simulink model "Robust_Adaptive_Control"  (R2015a)
settings: Solver=ode45  StartTime=0.0  StopTime=10  FixedStep=1e-3
libraries: aerolibutil x16, aerolibtransform2 x6, dspmtrx3 x6, simulink x1
(part 2 of 3)

== system Robust_Adaptive_Control/Slotine/u0-gen ==
  S : Inport
  sigma(t) : Inport  Port=2
  Divide : Product  Inputs=*/
  Dot Product : DotProduct  InputSameDT=on  OutDataTypeStr=Inherit: Inherit via internal rule
  Gain : Gain  Gain=-1
  Product : Product
  Product1 : Product
  Product2 : Product
  Sqrt : Sqrt  SaturateOnIntegerOverflow=on
  Sum : Sum  Inputs=|++
  gamma_hat : Integrator  InitialCondition=1
  u0 : Outport
  wires:
  gamma_hat/1 -> Product2/1, Product/2, Product/1
  Dot Product/1 -> Sqrt/1
  S/1 -> Product1/2, Dot Product/2, Dot Product/1
  Sqrt/1 -> Product2/2, gamma_hat/1
  Product/1 -> Product1/1
  Product1/1 -> Divide/1
  Product2/1 -> Sum/1
  Sum/1 -> Divide/2
  sigma(t)/1 -> Sum/2
  Divide/1 -> Gain/1
  Gain/1 -> u0/1

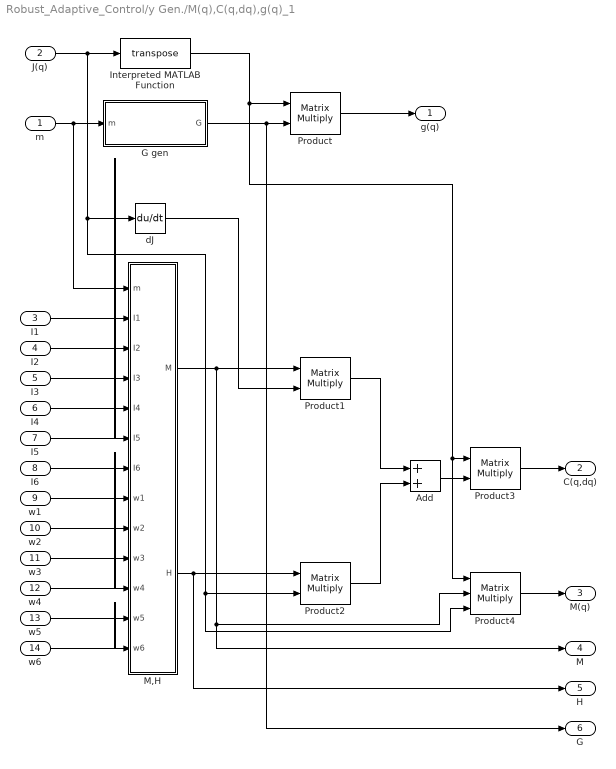
== system Robust_Adaptive_Control/y Gen./M(q),C(q,dq),g(q)_1 ==
  m : Inport
  J(q) : Inport  Port=2
  I1 : Inport  Port=3
  I2 : Inport  Port=4
  I3 : Inport  Port=5
  I4 : Inport  Port=6
  I5 : Inport  Port=7
  I6 : Inport  Port=8
  w1 : Inport  Port=9
  w2 : Inport  Port=10
  w3 : Inport  Port=11
  w4 : Inport  Port=12
  w5 : Inport  Port=13
  w6 : Inport  Port=14
  Add : Sum
  G gen : Subsystem
  Interpreted MATLAB Function : MATLABFcn  MATLABFcn=transpose  OutputSignalType=real  Output1D=off
  M,H : Subsystem
  Product{,1..3} (4 alike) : Product  Multiplication=Matrix(*)
  Product4 : Product  Inputs=3  Multiplication=Matrix(*)
  dJ : Derivative
  g(q) : Outport
  C(q,dq) : Outport  Port=2
  M(q) : Outport  Port=3
  M : Outport  Port=4
  H : Outport  Port=5
  G : Outport  Port=6
  wires:
  J(q)/1 -> Interpreted MATLAB Function/1, Product4/3, Product2/2, dJ/1
  Interpreted MATLAB Function/1 -> Product4/1, Product3/1, Product/1
  Product/1 -> g(q)/1
  m/1 -> M,H/1(m), G gen/1(m)
  I1/1 -> M,H/2(I1)
  I2/1 -> M,H/3(I2)
  I3/1 -> M,H/4(I3)
  I4/1 -> M,H/5(I4)
  I5/1 -> M,H/6(I5)
  I6/1 -> M,H/7(I6)
  w1/1 -> M,H/8(w1)
  w2/1 -> M,H/9(w2)
  w3/1 -> M,H/10(w3)
  w4/1 -> M,H/11(w4)
  w5/1 -> M,H/12(w5)
  w6/1 -> M,H/13(w6)
  M,H/1(M) -> Product1/1, M/1, Product4/2
  dJ/1 -> Product1/2
  M,H/2(H) -> H/1, Product2/1
  Product1/1 -> Add/1
  Product2/1 -> Add/2
  Add/1 -> Product3/2
  Product3/1 -> C(q,dq)/1
  Product4/1 -> M(q)/1
  G gen/1(G) -> G/1, Product/2

== system Robust_Adaptive_Control/y Gen./M(q),C(q,dq),g(q)_2 ==
  m : Inport
  J(q) : Inport  Port=2
  I1 : Inport  Port=3
  I2 : Inport  Port=4
  I3 : Inport  Port=5
  I4 : Inport  Port=6
  I5 : Inport  Port=7
  I6 : Inport  Port=8
  w1 : Inport  Port=9
  w2 : Inport  Port=10
  w3 : Inport  Port=11
  w4 : Inport  Port=12
  w5 : Inport  Port=13
  w6 : Inport  Port=14
  G gen : Subsystem
  Interpreted MATLAB Function : MATLABFcn  MATLABFcn=transpose  OutputSignalType=real  Output1D=off
  M,H : Subsystem
  Product : Product  Multiplication=Matrix(*)
  Product1 : Product  Multiplication=Matrix(*)
  Product3 : Product  Multiplication=Matrix(*)
  Product4 : Product  Inputs=3  Multiplication=Matrix(*)
  dJ : Derivative
  g(q) : Outport
  C(q,dq) : Outport  Port=2
  M(q) : Outport  Port=3
  M : Outport  Port=4
  H : Outport  Port=5
  G : Outport  Port=6
  wires:
  J(q)/1 -> Interpreted MATLAB Function/1, Product4/3, dJ/1
  Interpreted MATLAB Function/1 -> Product4/1, Product3/1, Product/1
  Product/1 -> g(q)/1
  m/1 -> G gen/1(m)
  I1/1 -> M,H/1(I1)
  I2/1 -> M,H/2(I2)
  I3/1 -> M,H/3(I3)
  I4/1 -> M,H/4(I4)
  I5/1 -> M,H/5(I5)
  I6/1 -> M,H/6(I6)
  w1/1 -> M,H/7(w1)
  w2/1 -> M,H/8(w2)
  w3/1 -> M,H/9(w3)
  w4/1 -> M,H/10(w4)
  w5/1 -> M,H/11(w5)
  w6/1 -> M,H/12(w6)
  M,H/1(M) -> Product1/1, M/1, Product4/2
  dJ/1 -> Product1/2
  M,H/2(H) -> H/1
  Product1/1 -> Product3/2
  Product3/1 -> C(q,dq)/1
  Product4/1 -> M(q)/1
  G gen/1(G) -> G/1, Product/2

== system Robust_Adaptive_Control/Jacobian/J(q) gen./J_v_1(q) ==
  Constant : Constant  Value=zeros(3,1)
  v2M_1 : MATLAB Function  TreatAsAtomicUnit=on
  v2M_2 : MATLAB Function  TreatAsAtomicUnit=on
  v2M_3 : MATLAB Function  TreatAsAtomicUnit=on
  v2M_4 : MATLAB Function  TreatAsAtomicUnit=on
  v2M_5 : MATLAB Function  TreatAsAtomicUnit=on
  J_v_1(q) : Outport
  wires:
  Constant/1 -> v2M_1/1(v1), v2M_5/2(v2), v2M_4/2(v2), v2M_3/2(v2), v2M_2/2(v2), v2M_1/2(v2)
  v2M_1/1(M) -> v2M_2/1(v1)
  v2M_2/1(M) -> v2M_3/1(v1)
  v2M_3/1(M) -> v2M_4/1(v1)
  v2M_4/1(M) -> v2M_5/1(v1)
  v2M_5/1(M) -> J_v_1(q)/1

== system Robust_Adaptive_Control/Jacobian/J(q) gen./J_v_2(q) ==
  R_1^0 : Inport
  p_1^0 : Inport  Port=2
  p_2^0 : Inport  Port=3
  type1 : Inport  Port=4
  Constant : Constant  Value=zeros(3,1)
  J_v_1 : Subsystem
  v2M_1 : MATLAB Function  TreatAsAtomicUnit=on
  v2M_2 : MATLAB Function  TreatAsAtomicUnit=on
  v2M_3 : MATLAB Function  TreatAsAtomicUnit=on
  v2M_4 : MATLAB Function  TreatAsAtomicUnit=on
  v2M_5 : MATLAB Function  TreatAsAtomicUnit=on
  J_v_2(q) : Outport
  wires:
  R_1^0/1 -> J_v_1/1(R)
  J_v_1/1(J_v) -> v2M_1/1(v1)
  v2M_1/1(M) -> v2M_2/1(v1)
  v2M_2/1(M) -> v2M_3/1(v1)
  v2M_3/1(M) -> v2M_4/1(v1)
  v2M_4/1(M) -> v2M_5/1(v1)
  v2M_5/1(M) -> J_v_2(q)/1
  Constant/1 -> v2M_3/2(v2), v2M_4/2(v2), v2M_5/2(v2), v2M_1/2(v2), v2M_2/2(v2)
  p_1^0/1 -> J_v_1/2(p)
  type1/1 -> J_v_1/4(type)
  p_2^0/1 -> J_v_1/3(pn)

== system Robust_Adaptive_Control/Jacobian/J(q) gen./J_v_3(q) ==
  R_1^0 : Inport
  R_2^0 : Inport  Port=2
  p_1^0 : Inport  Port=3
  p_2^0 : Inport  Port=4
  p_3^0 : Inport  Port=5
  type1 : Inport  Port=6
  type2 : Inport  Port=7
  Constant : Constant  Value=zeros(3,1)
  J_v_1 : Subsystem
  J_v_2 : Subsystem
  v2M_1 : MATLAB Function  TreatAsAtomicUnit=on
  v2M_2 : MATLAB Function  TreatAsAtomicUnit=on
  v2M_3 : MATLAB Function  TreatAsAtomicUnit=on
  v2M_4 : MATLAB Function  TreatAsAtomicUnit=on
  v2M_5 : MATLAB Function  TreatAsAtomicUnit=on
  J_v_3(q) : Outport
  wires:
  R_1^0/1 -> J_v_1/1(R)
  J_v_1/1(J_v) -> v2M_1/1(v1)
  v2M_1/1(M) -> v2M_2/1(v1)
  v2M_2/1(M) -> v2M_3/1(v1)
  v2M_3/1(M) -> v2M_4/1(v1)
  v2M_4/1(M) -> v2M_5/1(v1)
  v2M_5/1(M) -> J_v_3(q)/1
  J_v_2/1(J_v) -> v2M_1/2(v2)
  Constant/1 -> v2M_5/2(v2), v2M_4/2(v2), v2M_2/2(v2), v2M_3/2(v2)
  R_2^0/1 -> J_v_2/1(R)
  p_1^0/1 -> J_v_1/2(p)
  p_2^0/1 -> J_v_2/2(p)
  type2/1 -> J_v_2/4(type)
  type1/1 -> J_v_1/4(type)
  p_3^0/1 -> J_v_1/3(pn), J_v_2/3(pn)

== system Robust_Adaptive_Control/Jacobian/J(q) gen./J_v_4(q) ==
  R_1^0 : Inport
  R_2^0 : Inport  Port=2
  R_3^0 : Inport  Port=3
  p_1^0 : Inport  Port=4
  p_2^0 : Inport  Port=5
  p_3^0 : Inport  Port=6
  p_4^0 : Inport  Port=7
  type1 : Inport  Port=8
  type2 : Inport  Port=9
  type3 : Inport  Port=10
  Constant : Constant  Value=zeros(3,1)
  J_v_1 : Subsystem
  J_v_2 : Subsystem
  J_v_3 : Subsystem
  v2M_1 : MATLAB Function  TreatAsAtomicUnit=on
  v2M_2 : MATLAB Function  TreatAsAtomicUnit=on
  v2M_3 : MATLAB Function  TreatAsAtomicUnit=on
  v2M_4 : MATLAB Function  TreatAsAtomicUnit=on
  v2M_5 : MATLAB Function  TreatAsAtomicUnit=on
  J_v_4(q) : Outport
  wires:
  R_1^0/1 -> J_v_1/1(R)
  J_v_1/1(J_v) -> v2M_1/1(v1)
  v2M_1/1(M) -> v2M_2/1(v1)
  v2M_2/1(M) -> v2M_3/1(v1)
  v2M_3/1(M) -> v2M_4/1(v1)
  v2M_4/1(M) -> v2M_5/1(v1)
  v2M_5/1(M) -> J_v_4(q)/1
  J_v_2/1(J_v) -> v2M_1/2(v2)
  J_v_3/1(J_v) -> v2M_2/2(v2)
  Constant/1 -> v2M_5/2(v2), v2M_3/2(v2), v2M_4/2(v2)
  R_2^0/1 -> J_v_2/1(R)
  R_3^0/1 -> J_v_3/1(R)
  p_1^0/1 -> J_v_1/2(p)
  p_2^0/1 -> J_v_2/2(p)
  p_3^0/1 -> J_v_3/2(p)
  type2/1 -> J_v_2/4(type)
  type1/1 -> J_v_1/4(type)
  type3/1 -> J_v_3/4(type)
  p_4^0/1 -> J_v_1/3(pn), J_v_2/3(pn), J_v_3/3(pn)

== system Robust_Adaptive_Control/Jacobian/J(q) gen./J_v_5(q) ==
  R_1^0 : Inport
  R_2^0 : Inport  Port=2
  R_3^0 : Inport  Port=3
  R_4^0 : Inport  Port=4
  p_1^0 : Inport  Port=5
  p_2^0 : Inport  Port=6
  p_3^0 : Inport  Port=7
  p_4^0 : Inport  Port=8
  p_5^0 : Inport  Port=9
  type1 : Inport  Port=10
  type2 : Inport  Port=11
  type3 : Inport  Port=12
  type4 : Inport  Port=13
  Constant : Constant  Value=zeros(3,1)
  J_v_1 : Subsystem
  J_v_2 : Subsystem
  J_v_3 : Subsystem
  J_v_4 : Subsystem
  v2M_1 : MATLAB Function  TreatAsAtomicUnit=on
  v2M_2 : MATLAB Function  TreatAsAtomicUnit=on
  v2M_3 : MATLAB Function  TreatAsAtomicUnit=on
  v2M_4 : MATLAB Function  TreatAsAtomicUnit=on
  v2M_5 : MATLAB Function  TreatAsAtomicUnit=on
  J_v_5(q) : Outport
  wires:
  R_1^0/1 -> J_v_1/1(R)
  J_v_1/1(J_v) -> v2M_1/1(v1)
  v2M_1/1(M) -> v2M_2/1(v1)
  v2M_2/1(M) -> v2M_3/1(v1)
  v2M_3/1(M) -> v2M_4/1(v1)
  v2M_4/1(M) -> v2M_5/1(v1)
  v2M_5/1(M) -> J_v_5(q)/1
  J_v_2/1(J_v) -> v2M_1/2(v2)
  J_v_3/1(J_v) -> v2M_2/2(v2)
  J_v_4/1(J_v) -> v2M_3/2(v2)
  Constant/1 -> v2M_4/2(v2), v2M_5/2(v2)
  R_2^0/1 -> J_v_2/1(R)
  R_3^0/1 -> J_v_3/1(R)
  R_4^0/1 -> J_v_4/1(R)
  p_1^0/1 -> J_v_1/2(p)
  p_2^0/1 -> J_v_2/2(p)
  p_3^0/1 -> J_v_3/2(p)
  p_4^0/1 -> J_v_4/2(p)
  type2/1 -> J_v_2/4(type)
  type1/1 -> J_v_1/4(type)
  type3/1 -> J_v_3/4(type)
  type4/1 -> J_v_4/4(type)
  p_5^0/1 -> J_v_1/3(pn), J_v_2/3(pn), J_v_3/3(pn), J_v_4/3(pn)

== system Robust_Adaptive_Control/Jacobian/J_v/J_v_1 ==
  R : Inport
  p : Inport  Port=2
  pn : Inport  Port=3
  type : Inport  Port=4
  Add : Sum
  If : If  IfExpression=u1 == 1
  Prismatic Action : Subsystem  TreatAsAtomicUnit=on
  Revolute Action : Subsystem  TreatAsAtomicUnit=on
  J_v : Outport
  wires:
  type/1 -> If/1
  If/1 -> Revolute Action/Action
  If/2 -> Prismatic Action/Action
  Revolute Action/1(J_v) -> Add/1
  Prismatic Action/1(J_v) -> Add/2
  Add/1 -> J_v/1
  R/1 -> Prismatic Action/1(R), Revolute Action/1(R)
  p/1 -> Revolute Action/2(p)
  pn/1 -> Revolute Action/3(pn)

== system Robust_Adaptive_Control/Jacobian/J_v/J_v_2 ==
  R : Inport
  p : Inport  Port=2
  pn : Inport  Port=3
  type : Inport  Port=4
  Add : Sum
  If : If  IfExpression=u1 == 1
  Prismatic Action : Subsystem  TreatAsAtomicUnit=on
  Revolute Action : Subsystem  TreatAsAtomicUnit=on
  J_v : Outport
  wires:
  type/1 -> If/1
  If/1 -> Revolute Action/Action
  If/2 -> Prismatic Action/Action
  Revolute Action/1(J_v) -> Add/1
  Prismatic Action/1(J_v) -> Add/2
  Add/1 -> J_v/1
  R/1 -> Prismatic Action/1(R), Revolute Action/1(R)
  p/1 -> Revolute Action/2(p)
  pn/1 -> Revolute Action/3(pn)

== system Robust_Adaptive_Control/Jacobian/J_v/J_v_3 ==
  R : Inport
  p : Inport  Port=2
  pn : Inport  Port=3
  type : Inport  Port=4
  Add : Sum
  If : If  IfExpression=u1 == 1
  Prismatic Action : Subsystem  TreatAsAtomicUnit=on
  Revolute Action : Subsystem  TreatAsAtomicUnit=on
  J_v : Outport
  wires:
  type/1 -> If/1
  If/1 -> Revolute Action/Action
  If/2 -> Prismatic Action/Action
  Revolute Action/1(J_v) -> Add/1
  Prismatic Action/1(J_v) -> Add/2
  Add/1 -> J_v/1
  R/1 -> Prismatic Action/1(R), Revolute Action/1(R)
  p/1 -> Revolute Action/2(p)
  pn/1 -> Revolute Action/3(pn)

== system Robust_Adaptive_Control/Jacobian/J_v/J_v_4 ==
  R : Inport
  p : Inport  Port=2
  pn : Inport  Port=3
  type : Inport  Port=4
  Add : Sum
  If : If  IfExpression=u1 == 1
  Prismatic Action : Subsystem  TreatAsAtomicUnit=on
  Revolute Action : Subsystem  TreatAsAtomicUnit=on
  J_v : Outport
  wires:
  type/1 -> If/1
  If/1 -> Revolute Action/Action
  If/2 -> Prismatic Action/Action
  Revolute Action/1(J_v) -> Add/1
  Prismatic Action/1(J_v) -> Add/2
  Add/1 -> J_v/1
  R/1 -> Prismatic Action/1(R), Revolute Action/1(R)
  p/1 -> Revolute Action/2(p)
  pn/1 -> Revolute Action/3(pn)

== system Robust_Adaptive_Control/Jacobian/J_v/J_v_5 ==
  R : Inport
  p : Inport  Port=2
  pn : Inport  Port=3
  type : Inport  Port=4
  Add : Sum
  If : If  IfExpression=u1 == 1
  Prismatic Action : Subsystem  TreatAsAtomicUnit=on
  Revolute Action : Subsystem  TreatAsAtomicUnit=on
  J_v : Outport
  wires:
  type/1 -> If/1
  If/1 -> Revolute Action/Action
  If/2 -> Prismatic Action/Action
  Revolute Action/1(J_v) -> Add/1
  Prismatic Action/1(J_v) -> Add/2
  Add/1 -> J_v/1
  R/1 -> Prismatic Action/1(R), Revolute Action/1(R)
  p/1 -> Revolute Action/2(p)
  pn/1 -> Revolute Action/3(pn)

== system Robust_Adaptive_Control/Jacobian/J_v/J_v_6 ==
  R : Inport
  p : Inport  Port=2
  pn : Inport  Port=3
  type : Inport  Port=4
  Add : Sum
  If : If  IfExpression=u1 == 1
  Prismatic Action : Subsystem  TreatAsAtomicUnit=on
  Revolute Action : Subsystem  TreatAsAtomicUnit=on
  J_v : Outport
  wires:
  type/1 -> If/1
  If/1 -> Revolute Action/Action
  If/2 -> Prismatic Action/Action
  Revolute Action/1(J_v) -> Add/1
  Prismatic Action/1(J_v) -> Add/2
  Add/1 -> J_v/1
  R/1 -> Prismatic Action/1(R), Revolute Action/1(R)
  p/1 -> Revolute Action/2(p)
  pn/1 -> Revolute Action/3(pn)

== system Robust_Adaptive_Control/y Gen./M(q),C(q,dq),g(q)_1/G gen ==
  m : Inport
  Demux : Demux  Outputs=6
  Mux : Mux  Inputs=7
  Product{,1..5} (6 alike) : Product
  g : Constant  Value=[0;0;9.81]
  g1 : Constant  Value=zeros(18,1)
  G : Outport
  wires:
  m/1 -> Demux/1
  Demux/1 -> Product/1
  Demux/2 -> Product1/1
  Demux/3 -> Product2/1
  g/1 -> Product5/2, Product4/2, Product3/2, Product2/2, Product1/2, Product/2
  Demux/4 -> Product3/1
  Demux/5 -> Product4/1
  Demux/6 -> Product5/1
  Product1/1 -> Mux/2
  Product/1 -> Mux/1
  Product2/1 -> Mux/3
  Product4/1 -> Mux/5
  Product5/1 -> Mux/6
  Product3/1 -> Mux/4
  g1/1 -> Mux/7
  Mux/1 -> G/1

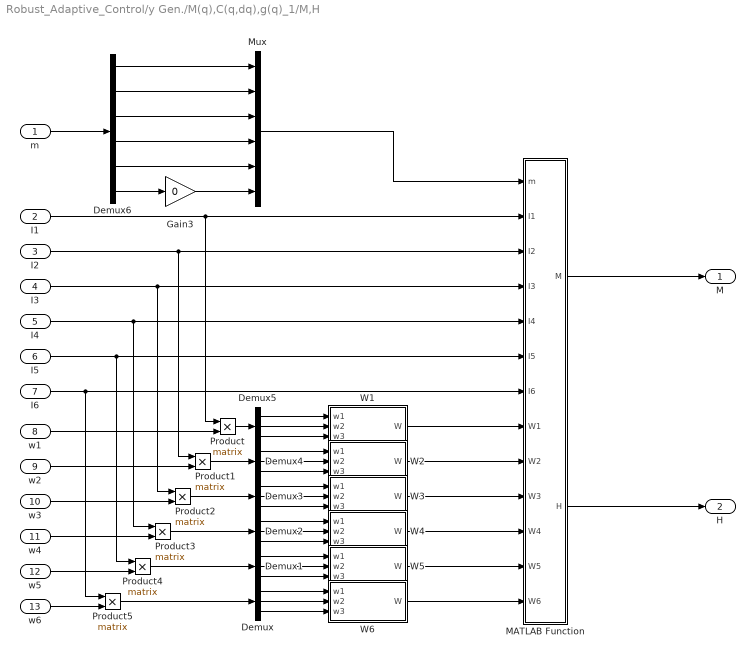
== system Robust_Adaptive_Control/y Gen./M(q),C(q,dq),g(q)_1/M,H ==
  m : Inport
  I1 : Inport  Port=2
  I2 : Inport  Port=3
  I3 : Inport  Port=4
  I4 : Inport  Port=5
  I5 : Inport  Port=6
  I6 : Inport  Port=7
  w1 : Inport  Port=8
  w2 : Inport  Port=9
  w3 : Inport  Port=10
  w4 : Inport  Port=11
  w5 : Inport  Port=12
  w6 : Inport  Port=13
  Demux{,1..5} (6 alike) : Demux  Outputs=3
  Demux6 : Demux  Outputs=6
  Gain3 : Gain  Gain=0
  MATLAB Function : MATLAB Function  TreatAsAtomicUnit=on
  Mux : Mux  Inputs=6
  Product{,1..5} (6 alike) : Product  Multiplication=Matrix(*)
  W1 : MATLAB Function  TreatAsAtomicUnit=on
  W2 : MATLAB Function  TreatAsAtomicUnit=on
  W3 : MATLAB Function  TreatAsAtomicUnit=on
  W4 : MATLAB Function  TreatAsAtomicUnit=on
  W5 : MATLAB Function  TreatAsAtomicUnit=on
  W6 : MATLAB Function  TreatAsAtomicUnit=on
  M : Outport
  H : Outport  Port=2
  wires:
  I1/1 -> Product/1, MATLAB Function/2(I1)
  I2/1 -> Product1/1, MATLAB Function/3(I2)
  I3/1 -> Product2/1, MATLAB Function/4(I3)
  I4/1 -> Product3/1, MATLAB Function/5(I4)
  I5/1 -> Product4/1, MATLAB Function/6(I5)
  I6/1 -> Product5/1, MATLAB Function/7(I6)
  MATLAB Function/1(M) -> M/1
  MATLAB Function/2(H) -> H/1
  W1/1(W) -> MATLAB Function/8(W1)
  W2/1(W) -> MATLAB Function/9(W2)
  W3/1(W) -> MATLAB Function/10(W3)
  W4/1(W) -> MATLAB Function/11(W4)
  W5/1(W) -> MATLAB Function/12(W5)
  W6/1(W) -> MATLAB Function/13(W6)
  w6/1 -> Product5/2
  Demux/3 -> W6/3(w3)
  Demux/2 -> W6/2(w2)
  Demux/1 -> W6/1(w1)
  w5/1 -> Product4/2
  Demux1/3 -> W5/3(w3)
  Demux1/2 -> W5/2(w2)
  Demux1/1 -> W5/1(w1)
  w4/1 -> Product3/2
  Demux2/3 -> W4/3(w3)
  Demux2/2 -> W4/2(w2)
  Demux2/1 -> W4/1(w1)
  w3/1 -> Product2/2
  Demux3/3 -> W3/3(w3)
  Demux3/2 -> W3/2(w2)
  Demux3/1 -> W3/1(w1)
  w2/1 -> Product1/2
  Demux4/3 -> W2/3(w3)
  Demux4/2 -> W2/2(w2)
  Demux4/1 -> W2/1(w1)
  w1/1 -> Product/2
  Demux5/3 -> W1/3(w3)
  Demux5/2 -> W1/2(w2)
  Demux5/1 -> W1/1(w1)
  Product/1 -> Demux5/1
  Product1/1 -> Demux4/1
  Product2/1 -> Demux3/1
  Product3/1 -> Demux2/1
  Product4/1 -> Demux1/1
  Product5/1 -> Demux/1
  m/1 -> Demux6/1
  Mux/1 -> MATLAB Function/1(m)
  Demux6/2 -> Mux/2
  Demux6/3 -> Mux/3
  Demux6/4 -> Mux/4
  Demux6/5 -> Mux/5
  Demux6/1 -> Mux/1
  Demux6/6 -> Gain3/1
  Gain3/1 -> Mux/6

== system Robust_Adaptive_Control/y Gen./M(q),C(q,dq),g(q)_2/G gen ==
  m : Inport
  Demux : Demux  Outputs=6
  Mux : Mux  Inputs=7
  Product{,1..5} (6 alike) : Product
  g : Constant  Value=[0;0;9.81]
  g1 : Constant  Value=zeros(18,1)
  G : Outport
  wires:
  m/1 -> Demux/1
  Demux/1 -> Product/1
  Demux/2 -> Product1/1
  Demux/3 -> Product2/1
  g/1 -> Product5/2, Product4/2, Product3/2, Product2/2, Product1/2, Product/2
  Demux/4 -> Product3/1
  Demux/5 -> Product4/1
  Demux/6 -> Product5/1
  Product1/1 -> Mux/2
  Product/1 -> Mux/1
  Product2/1 -> Mux/3
  Product4/1 -> Mux/5
  Product5/1 -> Mux/6
  Product3/1 -> Mux/4
  g1/1 -> Mux/7
  Mux/1 -> G/1

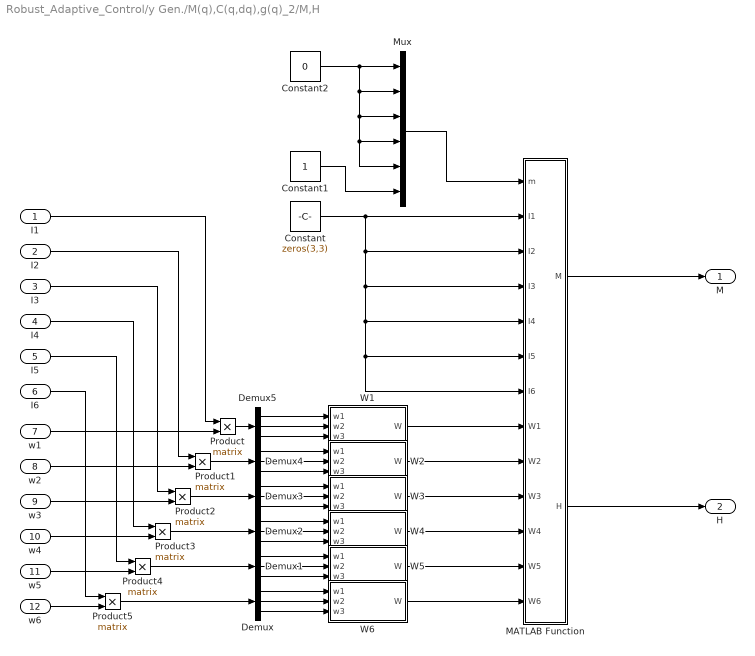
== system Robust_Adaptive_Control/y Gen./M(q),C(q,dq),g(q)_2/M,H ==
  I1 : Inport
  I2 : Inport  Port=2
  I3 : Inport  Port=3
  I4 : Inport  Port=4
  I5 : Inport  Port=5
  I6 : Inport  Port=6
  w1 : Inport  Port=7
  w2 : Inport  Port=8
  w3 : Inport  Port=9
  w4 : Inport  Port=10
  w5 : Inport  Port=11
  w6 : Inport  Port=12
  Constant : Constant  Value=zeros(3,3)
  Constant1 : Constant
  Constant2 : Constant  Value=0
  Demux{,1..5} (6 alike) : Demux  Outputs=3
  MATLAB Function : MATLAB Function  TreatAsAtomicUnit=on
  Mux : Mux  Inputs=6
  Product{,1..5} (6 alike) : Product  Multiplication=Matrix(*)
  W1 : MATLAB Function  TreatAsAtomicUnit=on
  W2 : MATLAB Function  TreatAsAtomicUnit=on
  W3 : MATLAB Function  TreatAsAtomicUnit=on
  W4 : MATLAB Function  TreatAsAtomicUnit=on
  W5 : MATLAB Function  TreatAsAtomicUnit=on
  W6 : MATLAB Function  TreatAsAtomicUnit=on
  M : Outport
  H : Outport  Port=2
  wires:
  I1/1 -> Product/1
  I2/1 -> Product1/1
  I3/1 -> Product2/1
  I4/1 -> Product3/1
  I5/1 -> Product4/1
  I6/1 -> Product5/1
  MATLAB Function/1(M) -> M/1
  MATLAB Function/2(H) -> H/1
  W1/1(W) -> MATLAB Function/8(W1)
  W2/1(W) -> MATLAB Function/9(W2)
  W3/1(W) -> MATLAB Function/10(W3)
  W4/1(W) -> MATLAB Function/11(W4)
  W5/1(W) -> MATLAB Function/12(W5)
  W6/1(W) -> MATLAB Function/13(W6)
  w6/1 -> Product5/2
  Demux/3 -> W6/3(w3)
  Demux/2 -> W6/2(w2)
  Demux/1 -> W6/1(w1)
  w5/1 -> Product4/2
  Demux1/3 -> W5/3(w3)
  Demux1/2 -> W5/2(w2)
  Demux1/1 -> W5/1(w1)
  w4/1 -> Product3/2
  Demux2/3 -> W4/3(w3)
  Demux2/2 -> W4/2(w2)
  Demux2/1 -> W4/1(w1)
  w3/1 -> Product2/2
  Demux3/3 -> W3/3(w3)
  Demux3/2 -> W3/2(w2)
  Demux3/1 -> W3/1(w1)
  w2/1 -> Product1/2
  Demux4/3 -> W2/3(w3)
  Demux4/2 -> W2/2(w2)
  Demux4/1 -> W2/1(w1)
  w1/1 -> Product/2
  Demux5/3 -> W1/3(w3)
  Demux5/2 -> W1/2(w2)
  Demux5/1 -> W1/1(w1)
  Product/1 -> Demux5/1
  Product1/1 -> Demux4/1
  Product2/1 -> Demux3/1
  Product3/1 -> Demux2/1
  Product4/1 -> Demux1/1
  Product5/1 -> Demux/1
  Mux/1 -> MATLAB Function/1(m)
  Constant/1 -> MATLAB Function/7(I6), MATLAB Function/6(I5), MATLAB Function/5(I4), MATLAB Function/4(I3), MATLAB Function/3(I2), MATLAB Function/2(I1)
  Constant1/1 -> Mux/6
  Constant2/1 -> Mux/3, Mux/5, Mux/4, Mux/2, Mux/1

== system Robust_Adaptive_Control/Jacobian/J(q) gen./J_v_2(q)/J_v_1 ==
  R : Inport
  p : Inport  Port=2
  pn : Inport  Port=3
  type : Inport  Port=4
  Add : Sum
  If : If  IfExpression=u1 == 1
  Prismatic Action : Subsystem  TreatAsAtomicUnit=on
  Revolute Action : Subsystem  TreatAsAtomicUnit=on
  J_v : Outport
  wires:
  type/1 -> If/1
  If/1 -> Revolute Action/Action
  If/2 -> Prismatic Action/Action
  Revolute Action/1(J_v) -> Add/1
  Prismatic Action/1(J_v) -> Add/2
  Add/1 -> J_v/1
  R/1 -> Prismatic Action/1(R), Revolute Action/1(R)
  p/1 -> Revolute Action/2(p)
  pn/1 -> Revolute Action/3(pn)

== system Robust_Adaptive_Control/Jacobian/J(q) gen./J_v_3(q)/J_v_1 ==
  R : Inport
  p : Inport  Port=2
  pn : Inport  Port=3
  type : Inport  Port=4
  Add : Sum
  If : If  IfExpression=u1 == 1
  Prismatic Action : Subsystem  TreatAsAtomicUnit=on
  Revolute Action : Subsystem  TreatAsAtomicUnit=on
  J_v : Outport
  wires:
  type/1 -> If/1
  If/1 -> Revolute Action/Action
  If/2 -> Prismatic Action/Action
  Revolute Action/1(J_v) -> Add/1
  Prismatic Action/1(J_v) -> Add/2
  Add/1 -> J_v/1
  R/1 -> Prismatic Action/1(R), Revolute Action/1(R)
  p/1 -> Revolute Action/2(p)
  pn/1 -> Revolute Action/3(pn)

== system Robust_Adaptive_Control/Jacobian/J(q) gen./J_v_3(q)/J_v_2 ==
  R : Inport
  p : Inport  Port=2
  pn : Inport  Port=3
  type : Inport  Port=4
  Add : Sum
  If : If  IfExpression=u1 == 1
  Prismatic Action : Subsystem  TreatAsAtomicUnit=on
  Revolute Action : Subsystem  TreatAsAtomicUnit=on
  J_v : Outport
  wires:
  type/1 -> If/1
  If/1 -> Revolute Action/Action
  If/2 -> Prismatic Action/Action
  Revolute Action/1(J_v) -> Add/1
  Prismatic Action/1(J_v) -> Add/2
  Add/1 -> J_v/1
  R/1 -> Prismatic Action/1(R), Revolute Action/1(R)
  p/1 -> Revolute Action/2(p)
  pn/1 -> Revolute Action/3(pn)

== system Robust_Adaptive_Control/Jacobian/J(q) gen./J_v_4(q)/J_v_1 ==
  R : Inport
  p : Inport  Port=2
  pn : Inport  Port=3
  type : Inport  Port=4
  Add : Sum
  If : If  IfExpression=u1 == 1
  Prismatic Action : Subsystem  TreatAsAtomicUnit=on
  Revolute Action : Subsystem  TreatAsAtomicUnit=on
  J_v : Outport
  wires:
  type/1 -> If/1
  If/1 -> Revolute Action/Action
  If/2 -> Prismatic Action/Action
  Revolute Action/1(J_v) -> Add/1
  Prismatic Action/1(J_v) -> Add/2
  Add/1 -> J_v/1
  R/1 -> Prismatic Action/1(R), Revolute Action/1(R)
  p/1 -> Revolute Action/2(p)
  pn/1 -> Revolute Action/3(pn)

== system Robust_Adaptive_Control/Jacobian/J(q) gen./J_v_4(q)/J_v_2 ==
  R : Inport
  p : Inport  Port=2
  pn : Inport  Port=3
  type : Inport  Port=4
  Add : Sum
  If : If  IfExpression=u1 == 1
  Prismatic Action : Subsystem  TreatAsAtomicUnit=on
  Revolute Action : Subsystem  TreatAsAtomicUnit=on
  J_v : Outport
  wires:
  type/1 -> If/1
  If/1 -> Revolute Action/Action
  If/2 -> Prismatic Action/Action
  Revolute Action/1(J_v) -> Add/1
  Prismatic Action/1(J_v) -> Add/2
  Add/1 -> J_v/1
  R/1 -> Prismatic Action/1(R), Revolute Action/1(R)
  p/1 -> Revolute Action/2(p)
  pn/1 -> Revolute Action/3(pn)

== system Robust_Adaptive_Control/Jacobian/J(q) gen./J_v_4(q)/J_v_3 ==
  R : Inport
  p : Inport  Port=2
  pn : Inport  Port=3
  type : Inport  Port=4
  Add : Sum
  If : If  IfExpression=u1 == 1
  Prismatic Action : Subsystem  TreatAsAtomicUnit=on
  Revolute Action : Subsystem  TreatAsAtomicUnit=on
  J_v : Outport
  wires:
  type/1 -> If/1
  If/1 -> Revolute Action/Action
  If/2 -> Prismatic Action/Action
  Revolute Action/1(J_v) -> Add/1
  Prismatic Action/1(J_v) -> Add/2
  Add/1 -> J_v/1
  R/1 -> Prismatic Action/1(R), Revolute Action/1(R)
  p/1 -> Revolute Action/2(p)
  pn/1 -> Revolute Action/3(pn)

== system Robust_Adaptive_Control/Jacobian/J(q) gen./J_v_5(q)/J_v_1 ==
  R : Inport
  p : Inport  Port=2
  pn : Inport  Port=3
  type : Inport  Port=4
  Add : Sum
  If : If  IfExpression=u1 == 1
  Prismatic Action : Subsystem  TreatAsAtomicUnit=on
  Revolute Action : Subsystem  TreatAsAtomicUnit=on
  J_v : Outport
  wires:
  type/1 -> If/1
  If/1 -> Revolute Action/Action
  If/2 -> Prismatic Action/Action
  Revolute Action/1(J_v) -> Add/1
  Prismatic Action/1(J_v) -> Add/2
  Add/1 -> J_v/1
  R/1 -> Prismatic Action/1(R), Revolute Action/1(R)
  p/1 -> Revolute Action/2(p)
  pn/1 -> Revolute Action/3(pn)

== system Robust_Adaptive_Control/Jacobian/J(q) gen./J_v_5(q)/J_v_2 ==
  R : Inport
  p : Inport  Port=2
  pn : Inport  Port=3
  type : Inport  Port=4
  Add : Sum
  If : If  IfExpression=u1 == 1
  Prismatic Action : Subsystem  TreatAsAtomicUnit=on
  Revolute Action : Subsystem  TreatAsAtomicUnit=on
  J_v : Outport
  wires:
  type/1 -> If/1
  If/1 -> Revolute Action/Action
  If/2 -> Prismatic Action/Action
  Revolute Action/1(J_v) -> Add/1
  Prismatic Action/1(J_v) -> Add/2
  Add/1 -> J_v/1
  R/1 -> Prismatic Action/1(R), Revolute Action/1(R)
  p/1 -> Revolute Action/2(p)
  pn/1 -> Revolute Action/3(pn)

== system Robust_Adaptive_Control/Jacobian/J(q) gen./J_v_5(q)/J_v_3 ==
  R : Inport
  p : Inport  Port=2
  pn : Inport  Port=3
  type : Inport  Port=4
  Add : Sum
  If : If  IfExpression=u1 == 1
  Prismatic Action : Subsystem  TreatAsAtomicUnit=on
  Revolute Action : Subsystem  TreatAsAtomicUnit=on
  J_v : Outport
  wires:
  type/1 -> If/1
  If/1 -> Revolute Action/Action
  If/2 -> Prismatic Action/Action
  Revolute Action/1(J_v) -> Add/1
  Prismatic Action/1(J_v) -> Add/2
  Add/1 -> J_v/1
  R/1 -> Prismatic Action/1(R), Revolute Action/1(R)
  p/1 -> Revolute Action/2(p)
  pn/1 -> Revolute Action/3(pn)

== system Robust_Adaptive_Control/Jacobian/J(q) gen./J_v_5(q)/J_v_4 ==
  R : Inport
  p : Inport  Port=2
  pn : Inport  Port=3
  type : Inport  Port=4
  Add : Sum
  If : If  IfExpression=u1 == 1
  Prismatic Action : Subsystem  TreatAsAtomicUnit=on
  Revolute Action : Subsystem  TreatAsAtomicUnit=on
  J_v : Outport
  wires:
  type/1 -> If/1
  If/1 -> Revolute Action/Action
  If/2 -> Prismatic Action/Action
  Revolute Action/1(J_v) -> Add/1
  Prismatic Action/1(J_v) -> Add/2
  Add/1 -> J_v/1
  R/1 -> Prismatic Action/1(R), Revolute Action/1(R)
  p/1 -> Revolute Action/2(p)
  pn/1 -> Revolute Action/3(pn)

== system Robust_Adaptive_Control/Jacobian/J_v/J_v_1/Prismatic Action ==
  R : Inport
  Action Port : ActionPort  ActionType=else
  Constant : Constant  Value=[0;0;1]
  Product : Product  Multiplication=Matrix(*)
  J_v : Outport
  wires:
  Product/1 -> J_v/1
  R/1 -> Product/1
  Constant/1 -> Product/2

== system Robust_Adaptive_Control/Jacobian/J_v/J_v_1/Revolute Action ==
  R : Inport
  p : Inport  Port=2
  pn : Inport  Port=3
  Action Port : ActionPort  ActionType=then
  3x3 Cross Product : aerolibutil/3x3 Cross Product
  Add : Sum  Inputs=-+
  Constant : Constant  Value=[0;0;1]
  Product : Product  Multiplication=Matrix(*)
  J_v : Outport
  wires:
  3x3 Cross Product/1 -> J_v/1
  p/1 -> Add/1
  pn/1 -> Add/2
  Add/1 -> 3x3 Cross Product/2
  R/1 -> Product/1
  Constant/1 -> Product/2
  Product/1 -> 3x3 Cross Product/1

== system Robust_Adaptive_Control/Jacobian/J_v/J_v_2/Prismatic Action ==
  R : Inport
  Action Port : ActionPort  ActionType=else
  Constant : Constant  Value=[0;0;1]
  Product : Product  Multiplication=Matrix(*)
  J_v : Outport
  wires:
  Product/1 -> J_v/1
  R/1 -> Product/1
  Constant/1 -> Product/2

== system Robust_Adaptive_Control/Jacobian/J_v/J_v_2/Revolute Action ==
  R : Inport
  p : Inport  Port=2
  pn : Inport  Port=3
  Action Port : ActionPort  ActionType=then
  3x3 Cross Product : aerolibutil/3x3 Cross Product
  Add : Sum  Inputs=-+
  Constant : Constant  Value=[0;0;1]
  Product : Product  Multiplication=Matrix(*)
  J_v : Outport
  wires:
  3x3 Cross Product/1 -> J_v/1
  p/1 -> Add/1
  pn/1 -> Add/2
  Add/1 -> 3x3 Cross Product/2
  R/1 -> Product/1
  Constant/1 -> Product/2
  Product/1 -> 3x3 Cross Product/1

== system Robust_Adaptive_Control/Jacobian/J_v/J_v_3/Prismatic Action ==
  R : Inport
  Action Port : ActionPort  ActionType=else
  Constant : Constant  Value=[0;0;1]
  Product : Product  Multiplication=Matrix(*)
  J_v : Outport
  wires:
  Product/1 -> J_v/1
  R/1 -> Product/1
  Constant/1 -> Product/2

== system Robust_Adaptive_Control/Jacobian/J_v/J_v_3/Revolute Action ==
  R : Inport
  p : Inport  Port=2
  pn : Inport  Port=3
  Action Port : ActionPort  ActionType=then
  3x3 Cross Product : aerolibutil/3x3 Cross Product
  Add : Sum  Inputs=-+
  Constant : Constant  Value=[0;0;1]
  Product : Product  Multiplication=Matrix(*)
  J_v : Outport
  wires:
  3x3 Cross Product/1 -> J_v/1
  p/1 -> Add/1
  pn/1 -> Add/2
  Add/1 -> 3x3 Cross Product/2
  R/1 -> Product/1
  Constant/1 -> Product/2
  Product/1 -> 3x3 Cross Product/1

== system Robust_Adaptive_Control/Jacobian/J_v/J_v_4/Prismatic Action ==
  R : Inport
  Action Port : ActionPort  ActionType=else
  Constant : Constant  Value=[0;0;1]
  Product : Product  Multiplication=Matrix(*)
  J_v : Outport
  wires:
  Product/1 -> J_v/1
  R/1 -> Product/1
  Constant/1 -> Product/2

== system Robust_Adaptive_Control/Jacobian/J_v/J_v_4/Revolute Action ==
  R : Inport
  p : Inport  Port=2
  pn : Inport  Port=3
  Action Port : ActionPort  ActionType=then
  3x3 Cross Product : aerolibutil/3x3 Cross Product
  Add : Sum  Inputs=-+
  Constant : Constant  Value=[0;0;1]
  Product : Product  Multiplication=Matrix(*)
  J_v : Outport
  wires:
  3x3 Cross Product/1 -> J_v/1
  p/1 -> Add/1
  pn/1 -> Add/2
  Add/1 -> 3x3 Cross Product/2
  R/1 -> Product/1
  Constant/1 -> Product/2
  Product/1 -> 3x3 Cross Product/1

== system Robust_Adaptive_Control/Jacobian/J_v/J_v_5/Prismatic Action ==
  R : Inport
  Action Port : ActionPort  ActionType=else
  Constant : Constant  Value=[0;0;1]
  Product : Product  Multiplication=Matrix(*)
  J_v : Outport
  wires:
  Product/1 -> J_v/1
  R/1 -> Product/1
  Constant/1 -> Product/2

== system Robust_Adaptive_Control/Jacobian/J_v/J_v_5/Revolute Action ==
  R : Inport
  p : Inport  Port=2
  pn : Inport  Port=3
  Action Port : ActionPort  ActionType=then
  3x3 Cross Product : aerolibutil/3x3 Cross Product
  Add : Sum  Inputs=-+
  Constant : Constant  Value=[0;0;1]
  Product : Product  Multiplication=Matrix(*)
  J_v : Outport
  wires:
  3x3 Cross Product/1 -> J_v/1
  p/1 -> Add/1
  pn/1 -> Add/2
  Add/1 -> 3x3 Cross Product/2
  R/1 -> Product/1
  Constant/1 -> Product/2
  Product/1 -> 3x3 Cross Product/1

== system Robust_Adaptive_Control/Jacobian/J_v/J_v_6/Prismatic Action ==
  R : Inport
  Action Port : ActionPort  ActionType=else
  Constant : Constant  Value=[0;0;1]
  Product : Product  Multiplication=Matrix(*)
  J_v : Outport
  wires:
  Product/1 -> J_v/1
  R/1 -> Product/1
  Constant/1 -> Product/2

== system Robust_Adaptive_Control/Jacobian/J_v/J_v_6/Revolute Action ==
  R : Inport
  p : Inport  Port=2
  pn : Inport  Port=3
  Action Port : ActionPort  ActionType=then
  3x3 Cross Product : aerolibutil/3x3 Cross Product
  Add : Sum  Inputs=-+
  Constant : Constant  Value=[0;0;1]
  Product : Product  Multiplication=Matrix(*)
  J_v : Outport
  wires:
  3x3 Cross Product/1 -> J_v/1
  p/1 -> Add/1
  pn/1 -> Add/2
  Add/1 -> 3x3 Cross Product/2
  R/1 -> Product/1
  Constant/1 -> Product/2
  Product/1 -> 3x3 Cross Product/1

== system Robust_Adaptive_Control/Jacobian/J(q) gen./J_v_2(q)/J_v_1/Prismatic Action ==
  R : Inport
  Action Port : ActionPort  ActionType=else
  Constant : Constant  Value=[0;0;1]
  Product : Product  Multiplication=Matrix(*)
  J_v : Outport
  wires:
  Product/1 -> J_v/1
  R/1 -> Product/1
  Constant/1 -> Product/2

== system Robust_Adaptive_Control/Jacobian/J(q) gen./J_v_2(q)/J_v_1/Revolute Action ==
  R : Inport
  p : Inport  Port=2
  pn : Inport  Port=3
  Action Port : ActionPort  ActionType=then
  3x3 Cross Product : aerolibutil/3x3 Cross Product
  Add : Sum  Inputs=-+
  Constant : Constant  Value=[0;0;1]
  Product : Product  Multiplication=Matrix(*)
  J_v : Outport
  wires:
  3x3 Cross Product/1 -> J_v/1
  p/1 -> Add/1
  pn/1 -> Add/2
  Add/1 -> 3x3 Cross Product/2
  R/1 -> Product/1
  Constant/1 -> Product/2
  Product/1 -> 3x3 Cross Product/1

== system Robust_Adaptive_Control/Jacobian/J(q) gen./J_v_3(q)/J_v_1/Prismatic Action ==
  R : Inport
  Action Port : ActionPort  ActionType=else
  Constant : Constant  Value=[0;0;1]
  Product : Product  Multiplication=Matrix(*)
  J_v : Outport
  wires:
  Product/1 -> J_v/1
  R/1 -> Product/1
  Constant/1 -> Product/2

== system Robust_Adaptive_Control/Jacobian/J(q) gen./J_v_3(q)/J_v_1/Revolute Action ==
  R : Inport
  p : Inport  Port=2
  pn : Inport  Port=3
  Action Port : ActionPort  ActionType=then
  3x3 Cross Product : aerolibutil/3x3 Cross Product
  Add : Sum  Inputs=-+
  Constant : Constant  Value=[0;0;1]
  Product : Product  Multiplication=Matrix(*)
  J_v : Outport
  wires:
  3x3 Cross Product/1 -> J_v/1
  p/1 -> Add/1
  pn/1 -> Add/2
  Add/1 -> 3x3 Cross Product/2
  R/1 -> Product/1
  Constant/1 -> Product/2
  Product/1 -> 3x3 Cross Product/1

== system Robust_Adaptive_Control/Jacobian/J(q) gen./J_v_3(q)/J_v_2/Prismatic Action ==
  R : Inport
  Action Port : ActionPort  ActionType=else
  Constant : Constant  Value=[0;0;1]
  Product : Product  Multiplication=Matrix(*)
  J_v : Outport
  wires:
  Product/1 -> J_v/1
  R/1 -> Product/1
  Constant/1 -> Product/2

== system Robust_Adaptive_Control/Jacobian/J(q) gen./J_v_3(q)/J_v_2/Revolute Action ==
  R : Inport
  p : Inport  Port=2
  pn : Inport  Port=3
  Action Port : ActionPort  ActionType=then
  3x3 Cross Product : aerolibutil/3x3 Cross Product
  Add : Sum  Inputs=-+
  Constant : Constant  Value=[0;0;1]
  Product : Product  Multiplication=Matrix(*)
  J_v : Outport
  wires:
  3x3 Cross Product/1 -> J_v/1
  p/1 -> Add/1
  pn/1 -> Add/2
  Add/1 -> 3x3 Cross Product/2
  R/1 -> Product/1
  Constant/1 -> Product/2
  Product/1 -> 3x3 Cross Product/1

== system Robust_Adaptive_Control/Jacobian/J(q) gen./J_v_4(q)/J_v_1/Prismatic Action ==
  R : Inport
  Action Port : ActionPort  ActionType=else
  Constant : Constant  Value=[0;0;1]
  Product : Product  Multiplication=Matrix(*)
  J_v : Outport
  wires:
  Product/1 -> J_v/1
  R/1 -> Product/1
  Constant/1 -> Product/2

== system Robust_Adaptive_Control/Jacobian/J(q) gen./J_v_4(q)/J_v_1/Revolute Action ==
  R : Inport
  p : Inport  Port=2
  pn : Inport  Port=3
  Action Port : ActionPort  ActionType=then
  3x3 Cross Product : aerolibutil/3x3 Cross Product
  Add : Sum  Inputs=-+
  Constant : Constant  Value=[0;0;1]
  Product : Product  Multiplication=Matrix(*)
  J_v : Outport
  wires:
  3x3 Cross Product/1 -> J_v/1
  p/1 -> Add/1
  pn/1 -> Add/2
  Add/1 -> 3x3 Cross Product/2
  R/1 -> Product/1
  Constant/1 -> Product/2
  Product/1 -> 3x3 Cross Product/1

== system Robust_Adaptive_Control/Jacobian/J(q) gen./J_v_4(q)/J_v_2/Prismatic Action ==
  R : Inport
  Action Port : ActionPort  ActionType=else
  Constant : Constant  Value=[0;0;1]
  Product : Product  Multiplication=Matrix(*)
  J_v : Outport
  wires:
  Product/1 -> J_v/1
  R/1 -> Product/1
  Constant/1 -> Product/2

== system Robust_Adaptive_Control/Jacobian/J(q) gen./J_v_4(q)/J_v_2/Revolute Action ==
  R : Inport
  p : Inport  Port=2
  pn : Inport  Port=3
  Action Port : ActionPort  ActionType=then
  3x3 Cross Product : aerolibutil/3x3 Cross Product
  Add : Sum  Inputs=-+
  Constant : Constant  Value=[0;0;1]
  Product : Product  Multiplication=Matrix(*)
  J_v : Outport
  wires:
  3x3 Cross Product/1 -> J_v/1
  p/1 -> Add/1
  pn/1 -> Add/2
  Add/1 -> 3x3 Cross Product/2
  R/1 -> Product/1
  Constant/1 -> Product/2
  Product/1 -> 3x3 Cross Product/1

== system Robust_Adaptive_Control/Jacobian/J(q) gen./J_v_4(q)/J_v_3/Prismatic Action ==
  R : Inport
  Action Port : ActionPort  ActionType=else
  Constant : Constant  Value=[0;0;1]
  Product : Product  Multiplication=Matrix(*)
  J_v : Outport
  wires:
  Product/1 -> J_v/1
  R/1 -> Product/1
  Constant/1 -> Product/2

== system Robust_Adaptive_Control/Jacobian/J(q) gen./J_v_4(q)/J_v_3/Revolute Action ==
  R : Inport
  p : Inport  Port=2
  pn : Inport  Port=3
  Action Port : ActionPort  ActionType=then
  3x3 Cross Product : aerolibutil/3x3 Cross Product
  Add : Sum  Inputs=-+
  Constant : Constant  Value=[0;0;1]
  Product : Product  Multiplication=Matrix(*)
  J_v : Outport
  wires:
  3x3 Cross Product/1 -> J_v/1
  p/1 -> Add/1
  pn/1 -> Add/2
  Add/1 -> 3x3 Cross Product/2
  R/1 -> Product/1
  Constant/1 -> Product/2
  Product/1 -> 3x3 Cross Product/1

== system Robust_Adaptive_Control/Jacobian/J(q) gen./J_v_5(q)/J_v_1/Prismatic Action ==
  R : Inport
  Action Port : ActionPort  ActionType=else
  Constant : Constant  Value=[0;0;1]
  Product : Product  Multiplication=Matrix(*)
  J_v : Outport
  wires:
  Product/1 -> J_v/1
  R/1 -> Product/1
  Constant/1 -> Product/2

== system Robust_Adaptive_Control/Jacobian/J(q) gen./J_v_5(q)/J_v_1/Revolute Action ==
  R : Inport
  p : Inport  Port=2
  pn : Inport  Port=3
  Action Port : ActionPort  ActionType=then
  3x3 Cross Product : aerolibutil/3x3 Cross Product
  Add : Sum  Inputs=-+
  Constant : Constant  Value=[0;0;1]
  Product : Product  Multiplication=Matrix(*)
  J_v : Outport
  wires:
  3x3 Cross Product/1 -> J_v/1
  p/1 -> Add/1
  pn/1 -> Add/2
  Add/1 -> 3x3 Cross Product/2
  R/1 -> Product/1
  Constant/1 -> Product/2
  Product/1 -> 3x3 Cross Product/1

== system Robust_Adaptive_Control/Jacobian/J(q) gen./J_v_5(q)/J_v_2/Prismatic Action ==
  R : Inport
  Action Port : ActionPort  ActionType=else
  Constant : Constant  Value=[0;0;1]
  Product : Product  Multiplication=Matrix(*)
  J_v : Outport
  wires:
  Product/1 -> J_v/1
  R/1 -> Product/1
  Constant/1 -> Product/2

== system Robust_Adaptive_Control/Jacobian/J(q) gen./J_v_5(q)/J_v_2/Revolute Action ==
  R : Inport
  p : Inport  Port=2
  pn : Inport  Port=3
  Action Port : ActionPort  ActionType=then
  3x3 Cross Product : aerolibutil/3x3 Cross Product
  Add : Sum  Inputs=-+
  Constant : Constant  Value=[0;0;1]
  Product : Product  Multiplication=Matrix(*)
  J_v : Outport
  wires:
  3x3 Cross Product/1 -> J_v/1
  p/1 -> Add/1
  pn/1 -> Add/2
  Add/1 -> 3x3 Cross Product/2
  R/1 -> Product/1
  Constant/1 -> Product/2
  Product/1 -> 3x3 Cross Product/1

== system Robust_Adaptive_Control/Jacobian/J(q) gen./J_v_5(q)/J_v_3/Prismatic Action ==
  R : Inport
  Action Port : ActionPort  ActionType=else
  Constant : Constant  Value=[0;0;1]
  Product : Product  Multiplication=Matrix(*)
  J_v : Outport
  wires:
  Product/1 -> J_v/1
  R/1 -> Product/1
  Constant/1 -> Product/2

== system Robust_Adaptive_Control/Jacobian/J(q) gen./J_v_5(q)/J_v_3/Revolute Action ==
  R : Inport
  p : Inport  Port=2
  pn : Inport  Port=3
  Action Port : ActionPort  ActionType=then
  3x3 Cross Product : aerolibutil/3x3 Cross Product
  Add : Sum  Inputs=-+
  Constant : Constant  Value=[0;0;1]
  Product : Product  Multiplication=Matrix(*)
  J_v : Outport
  wires:
  3x3 Cross Product/1 -> J_v/1
  p/1 -> Add/1
  pn/1 -> Add/2
  Add/1 -> 3x3 Cross Product/2
  R/1 -> Product/1
  Constant/1 -> Product/2
  Product/1 -> 3x3 Cross Product/1

== system Robust_Adaptive_Control/Jacobian/J(q) gen./J_v_5(q)/J_v_4/Prismatic Action ==
  R : Inport
  Action Port : ActionPort  ActionType=else
  Constant : Constant  Value=[0;0;1]
  Product : Product  Multiplication=Matrix(*)
  J_v : Outport
  wires:
  Product/1 -> J_v/1
  R/1 -> Product/1
  Constant/1 -> Product/2

== system Robust_Adaptive_Control/Jacobian/J(q) gen./J_v_5(q)/J_v_4/Revolute Action ==
  R : Inport
  p : Inport  Port=2
  pn : Inport  Port=3
  Action Port : ActionPort  ActionType=then
  3x3 Cross Product : aerolibutil/3x3 Cross Product
  Add : Sum  Inputs=-+
  Constant : Constant  Value=[0;0;1]
  Product : Product  Multiplication=Matrix(*)
  J_v : Outport
  wires:
  3x3 Cross Product/1 -> J_v/1
  p/1 -> Add/1
  pn/1 -> Add/2
  Add/1 -> 3x3 Cross Product/2
  R/1 -> Product/1
  Constant/1 -> Product/2
  Product/1 -> 3x3 Cross Product/1

== matlab function Robust_Adaptive_Control/H_6^0/H_5^4/MATLAB Function ==
  data: R input; H output; p input
function H = fcn(R,p)

H = [R          p
     zeros(1,3) 1];

== matlab function Robust_Adaptive_Control/H_6^0/H_4^3/MATLAB Function ==
  data: R input; H output; p input
function H = fcn(R,p)

H = [R          p
     zeros(1,3) 1];

== matlab function Robust_Adaptive_Control/H_6^0/H_3^2/MATLAB Function ==
  data: R input; H output; p input
function H = fcn(R,p)

H = [R          p
     zeros(1,3) 1];

== matlab function Robust_Adaptive_Control/H_6^0/H_2^1/MATLAB Function ==
  data: R input; H output; p input
function H = fcn(R,p)

H = [R          p
     zeros(1,3) 1];

== matlab function Robust_Adaptive_Control/H_6^0/H_1^0/MATLAB Function ==
  data: R input; H output; p input
function H = fcn(R,p)

H = [R          p
     zeros(1,3) 1];

== matlab function Robust_Adaptive_Control/Jacobian/J(q) gen./J_v_1(q)/v2M_1 ==
  data: v1 input; M output; v2 input
function M = fcn(v1,v2)

M=[v1 v2];

== matlab function Robust_Adaptive_Control/Jacobian/J_w/J_w_1 ==
  data: R input; J_w output; type input
function J_w = fcn(R,type)

if type==1
    
    J_w=R*[0;0;1];
    
else
    
    J_w=zeros(3,1);
    
end

== matlab function Robust_Adaptive_Control/H_6^0/H_6^5/MATLAB Function ==
  data: R input; H output; p input
function H = fcn(R,p)

H = [R          p
     zeros(1,3) 1];

== matlab function Robust_Adaptive_Control/Jacobian/J_w/J_w_2 ==
  data: R input; J_w output; type input
function J_w = fcn(R,type)

if type==1
    
    J_w=R*[0;0;1];
    
else
    
    J_w=zeros(3,1);
    
end

== matlab function Robust_Adaptive_Control/Jacobian/J_w/J_w_3 ==
  data: R input; J_w output; type input
function J_w = fcn(R,type)

if type==1
    
    J_w=R*[0;0;1];
    
else
    
    J_w=zeros(3,1);
    
end

== matlab function Robust_Adaptive_Control/Jacobian/J_w/J_w_4 ==
  data: R input; J_w output; type input
function J_w = fcn(R,type)

if type==1
    
    J_w=R*[0;0;1];
    
else
    
    J_w=zeros(3,1);
    
end

== matlab function Robust_Adaptive_Control/Jacobian/J_w/J_w_5 ==
  data: R input; J_w output; type input
function J_w = fcn(R,type)

if type==1
    
    J_w=R*[0;0;1];
    
else
    
    J_w=zeros(3,1);
    
end

== matlab function Robust_Adaptive_Control/Jacobian/J_w/J_w_6 ==
  data: R input; J_w output; type input
function J_w = fcn(R,type)

if type==1
    
    J_w=R*[0;0;1];
    
else
    
    J_w=zeros(3,1);
    
end

== matlab function Robust_Adaptive_Control/Jacobian/J_w/v2M_1 ==
  data: v1 input; M output; v2 input
function M = fcn(v1,v2)

M=[v1 v2];

== matlab function Robust_Adaptive_Control/Jacobian/J_w/v2M_2 ==
  data: v1 input; M output; v2 input
function M = fcn(v1,v2)

M=[v1 v2];

== matlab function Robust_Adaptive_Control/Jacobian/J_w/v2M_3 ==
  data: v1 input; M output; v2 input
function M = fcn(v1,v2)

M=[v1 v2];

== matlab function Robust_Adaptive_Control/Jacobian/J_w/v2M_4 ==
  data: v1 input; M output; v2 input
function M = fcn(v1,v2)

M=[v1 v2];

== matlab function Robust_Adaptive_Control/Jacobian/J_w/v2M_5 ==
  data: v1 input; M output; v2 input
function M = fcn(v1,v2)

M=[v1 v2];

== matlab function Robust_Adaptive_Control/Jacobian/J(q) gen./J_v_1(q)/v2M_2 ==
  data: v1 input; M output; v2 input
function M = fcn(v1,v2)

M=[v1 v2];

== matlab function Robust_Adaptive_Control/Jacobian/J(q) gen./J_v_1(q)/v2M_3 ==
  data: v1 input; M output; v2 input
function M = fcn(v1,v2)

M=[v1 v2];

== matlab function Robust_Adaptive_Control/Jacobian/J(q) gen./J_v_1(q)/v2M_4 ==
  data: v1 input; M output; v2 input
function M = fcn(v1,v2)

M=[v1 v2];

== matlab function Robust_Adaptive_Control/Jacobian/J(q) gen./J_v_1(q)/v2M_5 ==
  data: v1 input; M output; v2 input
function M = fcn(v1,v2)

M=[v1 v2];

== matlab function Robust_Adaptive_Control/Jacobian/J(q) gen./J_v_2(q)/v2M_1 ==
  data: v1 input; M output; v2 input
function M = fcn(v1,v2)

M=[v1 v2];

== matlab function Robust_Adaptive_Control/Jacobian/J(q) gen./J_v_2(q)/v2M_2 ==
  data: v1 input; M output; v2 input
function M = fcn(v1,v2)

M=[v1 v2];

== matlab function Robust_Adaptive_Control/Jacobian/J_v/v2M_1 ==
  data: v1 input; M output; v2 input
function M = fcn(v1,v2)

M=[v1 v2];

== matlab function Robust_Adaptive_Control/Jacobian/J_v/v2M_2 ==
  data: v1 input; M output; v2 input
function M = fcn(v1,v2)

M=[v1 v2];

== matlab function Robust_Adaptive_Control/Jacobian/J_v/v2M_3 ==
  data: v1 input; M output; v2 input
function M = fcn(v1,v2)

M=[v1 v2];

== matlab function Robust_Adaptive_Control/Jacobian/J_v/v2M_4 ==
  data: v1 input; M output; v2 input
function M = fcn(v1,v2)

M=[v1 v2];

== matlab function Robust_Adaptive_Control/Jacobian/J_v/v2M_5 ==
  data: v1 input; M output; v2 input
function M = fcn(v1,v2)

M=[v1 v2];

== matlab function Robust_Adaptive_Control/M(q),C(q,dq),g(q)/M,H/MATLAB Function ==
  data: m input; M output; I1 input; I2 input; I3 input; I4 input; I5 input; I6 input; W1 input; W2 input; W3 input; W4 input; W5 input; W6 input; H output
function [M,H] = fcn(m,I1,I2,I3,I4,I5,I6,W1,W2,W3,W4,W5,W6)
%#codegen

M = blkdiag(m(1)*eye(3),m(2)*eye(3),m(3)*eye(3),m(4)*eye(3),m(5)*eye(3),m(6)*eye(3),...
            I1,I2,I3,I4,I5,I6);

H =-blkdiag(zeros(18,18),W1,W2,W3,W4,W5,W6);

== matlab function Robust_Adaptive_Control/M(q),C(q,dq),g(q)/M,H/W1 ==
  data: w1 input; W output; w2 input; w3 input
function W = fcn(w1,w2,w3)

W = [0    -w3  w2
     w3    0  -w1
    -w2    w1  0];

== matlab function Robust_Adaptive_Control/M(q),C(q,dq),g(q)/M,H/W2 ==
  data: w1 input; W output; w2 input; w3 input
function W = fcn(w1,w2,w3)

W = [0    -w3  w2
     w3  0    -w1
    -w2  w1  0];

== matlab function Robust_Adaptive_Control/M(q),C(q,dq),g(q)/M,H/W3 ==
  data: w1 input; W output; w2 input; w3 input
function W = fcn(w1,w2,w3)

W = [0    -w3  w2
     w3  0    -w1
    -w2  w1  0];

== matlab function Robust_Adaptive_Control/M(q),C(q,dq),g(q)/M,H/W4 ==
  data: w1 input; W output; w2 input; w3 input
function W = fcn(w1,w2,w3)

W = [0    -w3  w2
     w3  0    -w1
    -w2  w1  0];

== matlab function Robust_Adaptive_Control/M(q),C(q,dq),g(q)/M,H/W5 ==
  data: w1 input; W output; w2 input; w3 input
function W = fcn(w1,w2,w3)

W = [0    -w3  w2
     w3  0    -w1
    -w2  w1  0];

== matlab function Robust_Adaptive_Control/M(q),C(q,dq),g(q)/M,H/W6 ==
  data: w1 input; W output; w2 input; w3 input
function W = fcn(w1,w2,w3)

W = [0    -w3  w2
     w3  0    -w1
    -w2  w1  0];

== matlab function Robust_Adaptive_Control/Jacobian/J(q) gen./J_v_2(q)/v2M_3 ==
  data: v1 input; M output; v2 input
function M = fcn(v1,v2)

M=[v1 v2];

== matlab function Robust_Adaptive_Control/Jacobian/J(q) gen./J_v_2(q)/v2M_4 ==
  data: v1 input; M output; v2 input
function M = fcn(v1,v2)

M=[v1 v2];

== matlab function Robust_Adaptive_Control/Jacobian/J(q) gen./J_v_2(q)/v2M_5 ==
  data: v1 input; M output; v2 input
function M = fcn(v1,v2)

M=[v1 v2];

== matlab function Robust_Adaptive_Control/Jacobian/J(q) gen./J_v_3(q)/v2M_1 ==
  data: v1 input; M output; v2 input
function M = fcn(v1,v2)

M=[v1 v2];

== matlab function Robust_Adaptive_Control/Jacobian/J(q) gen./J_v_3(q)/v2M_2 ==
  data: v1 input; M output; v2 input
function M = fcn(v1,v2)

M=[v1 v2];

== matlab function Robust_Adaptive_Control/Jacobian/J(q) gen./J_v_3(q)/v2M_3 ==
  data: v1 input; M output; v2 input
function M = fcn(v1,v2)

M=[v1 v2];

== matlab function Robust_Adaptive_Control/Jacobian/J(q) gen./J_v_3(q)/v2M_4 ==
  data: v1 input; M output; v2 input
function M = fcn(v1,v2)

M=[v1 v2];

== matlab function Robust_Adaptive_Control/Jacobian/J(q) gen./J_v_3(q)/v2M_5 ==
  data: v1 input; M output; v2 input
function M = fcn(v1,v2)

M=[v1 v2];

== matlab function Robust_Adaptive_Control/Jacobian/J(q) gen./J_v_4(q)/v2M_1 ==
  data: v1 input; M output; v2 input
function M = fcn(v1,v2)

M=[v1 v2];

== matlab function Robust_Adaptive_Control/Jacobian/J(q) gen./J_v_4(q)/v2M_2 ==
  data: v1 input; M output; v2 input
function M = fcn(v1,v2)

M=[v1 v2];

== matlab function Robust_Adaptive_Control/Jacobian/J(q) gen./J_v_4(q)/v2M_3 ==
  data: v1 input; M output; v2 input
function M = fcn(v1,v2)

M=[v1 v2];

== matlab function Robust_Adaptive_Control/Jacobian/J(q) gen./J_v_4(q)/v2M_4 ==
  data: v1 input; M output; v2 input
function M = fcn(v1,v2)

M=[v1 v2];

== matlab function Robust_Adaptive_Control/Jacobian/J(q) gen./J_v_4(q)/v2M_5 ==
  data: v1 input; M output; v2 input
function M = fcn(v1,v2)

M=[v1 v2];

== matlab function Robust_Adaptive_Control/Jacobian/J(q) gen./J_v_5(q)/v2M_1 ==
  data: v1 input; M output; v2 input
function M = fcn(v1,v2)

M=[v1 v2];

== matlab function Robust_Adaptive_Control/Jacobian/J(q) gen./J_v_5(q)/v2M_2 ==
  data: v1 input; M output; v2 input
function M = fcn(v1,v2)

M=[v1 v2];

== matlab function Robust_Adaptive_Control/Jacobian/J(q) gen./J_v_5(q)/v2M_3 ==
  data: v1 input; M output; v2 input
function M = fcn(v1,v2)

M=[v1 v2];

== matlab function Robust_Adaptive_Control/Jacobian/J(q) gen./J_v_5(q)/v2M_4 ==
  data: v1 input; M output; v2 input
function M = fcn(v1,v2)

M=[v1 v2];

== matlab function Robust_Adaptive_Control/Jacobian/J(q) gen./J_v_5(q)/v2M_5 ==
  data: v1 input; M output; v2 input
function M = fcn(v1,v2)

M=[v1 v2];

== matlab function Robust_Adaptive_Control/Jacobian/J(q) gen./MATLAB Function ==
  data: J_w1 input; J_q output; J_w2 input; J_w3 input; J_w4 input; J_w5 input; J_w6 input; J_v1 input; J_v2 input; J_v3 input; J_v4 input; J_v5 input; J_v6 input; R1 input; R2 input; R3 input; R4 input; R5 input; R6 input
function J_q = fcn(J_w1,J_w2,J_w3,J_w4,J_w5,J_w6,J_v1,J_v2,J_v3,J_v4,J_v5,J_v6,R1,R2,R3,R4,R5,R6)


J_q=[J_v1
     J_v2
     J_v3
     J_v4
     J_v5
     J_v6
     R1'*J_w1 zeros(3,5)
     R2'*J_w1 R2'*J_w2 zeros(3,4)
     R3'*J_w1 R3'*J_w2 R3'*J_w3 zeros(3,3)
     R4'*J_w1 R4'*J_w2 R4'*J_w3 R4'*J_w4 zeros(3,2)
     R5'*J_w1 R5'*J_w2 R5'*J_w3 R5'*J_w4 R5'*J_w5 zeros(3,1)
     R6'*J_w1 R6'*J_w2 R6'*J_w3 R6'*J_w4 R6'*J_w5 R6'*J_w6];

== matlab function Robust_Adaptive_Control/y Gen./M(q),C(q,dq),g(q)_1/M,H/MATLAB Function ==
  data: m input; M output; I1 input; I2 input; I3 input; I4 input; I5 input; I6 input; W1 input; W2 input; W3 input; W4 input; W5 input; W6 input; H output
function [M,H] = fcn(m,I1,I2,I3,I4,I5,I6,W1,W2,W3,W4,W5,W6)
%#codegen

M = blkdiag(m(1)*eye(3),m(2)*eye(3),m(3)*eye(3),m(4)*eye(3),m(5)*eye(3),m(6)*eye(3),...
            I1,I2,I3,I4,I5,I6);

H =-blkdiag(zeros(18,18),W1,W2,W3,W4,W5,W6);

== matlab function Robust_Adaptive_Control/y Gen./M(q),C(q,dq),g(q)_1/M,H/W1 ==
  data: w1 input; W output; w2 input; w3 input
function W = fcn(w1,w2,w3)

W = [0    -w3  w2
     w3    0  -w1
    -w2    w1  0];

== matlab function Robust_Adaptive_Control/y Gen./M(q),C(q,dq),g(q)_1/M,H/W2 ==
  data: w1 input; W output; w2 input; w3 input
function W = fcn(w1,w2,w3)

W = [0    -w3  w2
     w3  0    -w1
    -w2  w1  0];

== matlab function Robust_Adaptive_Control/y Gen./M(q),C(q,dq),g(q)_1/M,H/W3 ==
  data: w1 input; W output; w2 input; w3 input
function W = fcn(w1,w2,w3)

W = [0    -w3  w2
     w3  0    -w1
    -w2  w1  0];

== matlab function Robust_Adaptive_Control/y Gen./M(q),C(q,dq),g(q)_1/M,H/W4 ==
  data: w1 input; W output; w2 input; w3 input
function W = fcn(w1,w2,w3)

W = [0    -w3  w2
     w3  0    -w1
    -w2  w1  0];

== matlab function Robust_Adaptive_Control/y Gen./M(q),C(q,dq),g(q)_1/M,H/W5 ==
  data: w1 input; W output; w2 input; w3 input
function W = fcn(w1,w2,w3)

W = [0    -w3  w2
     w3  0    -w1
    -w2  w1  0];
